simulink model "mrefrobotarm_modified_previous_y_previous_u_previous_ref_Thao"  (R2018b)
settings: Solver=FixedStepAuto  StartTime=0.0  StopTime=10  RelTol=1e-3  AbsTol=1e-6
undefined symbols (not defined in the file or in its folder): sfunxy2
libraries: neural x668, simulink x1
(part 11 of 21)

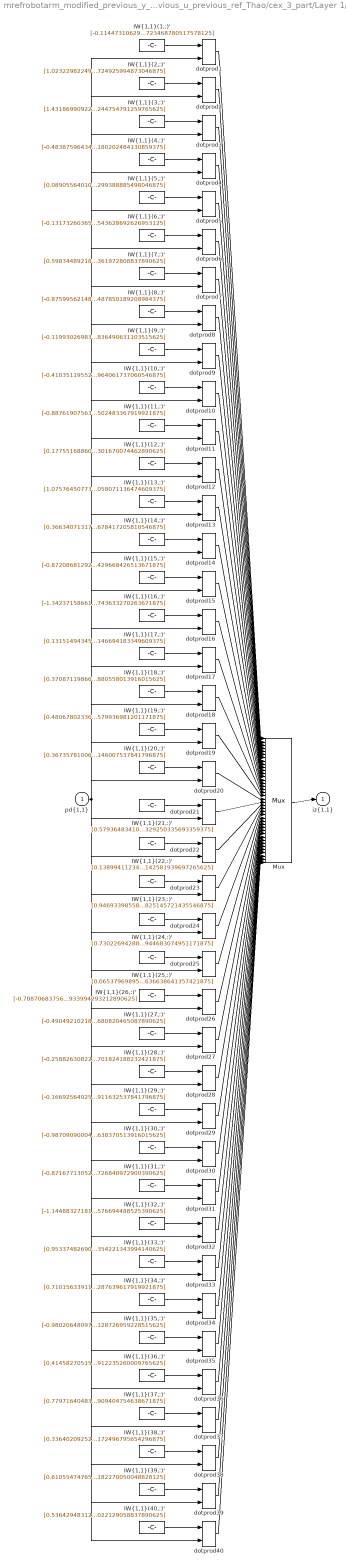
== system mrefrobotarm_modified_previous_y_previous_u_previous_ref_Thao/cex_3_part/Layer 1/IW{1,1} ==
  "pd{1,1}" : Inport  PortDimensions=10
      mask Display: e = 0.06;c1 = [120 230 180]/255;c2 = ([120 230 180]+0)/(256+128);c3 = ([120 230 180]+128)/(256+128);patch([0 1 1 0],[0 0 1 1],c1);patch([0 1 1 1-e 1-e 0+e],[0 0 1 1-e 0+e 0+e],c2);patch([0 0 1 1-e 0+e 0+e],[0 1 1 1-e 1-e 0+e],c3);plot([0 1 1 0 0],[0 0 1 1 0]);
  "IW{1,1}(1,:)'" : Constant  Value=[-0.11447310629155120487165930853734607808291912078857421875;1.4698726288777439474841912669944576919078826904296875;-0.1723351665624642536922550561939715407788753509521484375;0.06363633275744169648380221815386903472244739532470703125;-0.5064381225659226881674612741335295140743255615234375;-0.87026544298500951857278096213121898472309112548828125;-0.05463414776289564345201910100513487122952938079833984375;-1.13665173088892235142566278227604925632476806640625;0.268135298745105721263115583496983163058757781982421875;0.80221792322600216085248803210561163723468780517578125]
      mask Display: e = 0.06;c1 = [120 150 230]/255;c2 = ([120 150 230]+0)/383;c3 = ([120 150 230]+128)/383;patch([0 1 1 0],[0 0 1 1],c1);patch([0 1 1 1-e 1-e 0+e],[0 0 1 1-e 0+e 0+e],c2);patch([0 0 1 1-e 0+e 0+e],[0 1 1 1-e 1-e 0+e],c3);plot([0 1 1 0 0],[0 0 1 1 0]);disp('Weights');
  "IW{1,1}(10,:)'" : Constant  Value=[-0.41035119552119725394589977440773509442806243896484375;0.379787039117026992141035179884056560695171356201171875;-0.6683306949706373512043455775710754096508026123046875;-0.554820790867510016397545768995769321918487548828125;-0.71829482967000668480750391609035432338714599609375;0.447818372430159594710374904025229625403881072998046875;-0.55799752266937974187754889499046839773654937744140625;-0.379991668177938557438011457634274847805500030517578125;-0.340403705678418655455885755145573057234287261962890625;0.8973758576824291122164822809281758964061737060546875]
      mask Display: e = 0.06;c1 = [120 150 230]/255;c2 = ([120 150 230]+0)/383;c3 = ([120 150 230]+128)/383;patch([0 1 1 0],[0 0 1 1],c1);patch([0 1 1 1-e 1-e 0+e],[0 0 1 1-e 0+e 0+e],c2);patch([0 0 1 1-e 0+e 0+e],[0 1 1 1-e 1-e 0+e],c3);plot([0 1 1 0 0],[0 0 1 1 0]);disp('Weights');
  "IW{1,1}(11,:)'" : Constant  Value=[-0.8876190756363431244579942358541302382946014404296875;-1.025355338770573165874111509765498340129852294921875;0.1069134658050685526831102833966724574565887451171875;0.97378772065178031969168159776018001139163970947265625;-0.499558978367755146532402932280092500150203704833984375;-0.6707411879199665083461923131835646927356719970703125;-0.45046584360111163736206663088523782789707183837890625;0.415682749022733333266188537891139276325702667236328125;0.50981038413725221492001082879141904413700103759765625;-0.1924767238865232321654019642664934508502483367919921875]
      mask Display: e = 0.06;c1 = [120 150 230]/255;c2 = ([120 150 230]+0)/383;c3 = ([120 150 230]+128)/383;patch([0 1 1 0],[0 0 1 1],c1);patch([0 1 1 1-e 1-e 0+e],[0 0 1 1-e 0+e 0+e],c2);patch([0 0 1 1-e 0+e 0+e],[0 1 1 1-e 1-e 0+e],c3);plot([0 1 1 0 0],[0 0 1 1 0]);disp('Weights');
  "IW{1,1}(12,:)'" : Constant  Value=[0.177551688602920088033698675644700415432453155517578125;0.59145549863474300433807684385101310908794403076171875;-0.9027361748370814620301416653092019259929656982421875;0.70169416622816183082278485017013736069202423095703125;0.2632759672114854954116935914498753845691680908203125;0.392263699137575139186395745127811096608638763427734375;-0.444286429846018904310511743460665456950664520263671875;0.81245600109735327531979010018403641879558563232421875;-0.125222673969303255336882330084335990250110626220703125;0.0723812960570092978063172495239996351301670074462890625]
      mask Display: e = 0.06;c1 = [120 150 230]/255;c2 = ([120 150 230]+0)/383;c3 = ([120 150 230]+128)/383;patch([0 1 1 0],[0 0 1 1],c1);patch([0 1 1 1-e 1-e 0+e],[0 0 1 1-e 0+e 0+e],c2);patch([0 0 1 1-e 0+e 0+e],[0 1 1 1-e 1-e 0+e],c3);plot([0 1 1 0 0],[0 0 1 1 0]);disp('Weights');
  "IW{1,1}(13,:)'" : Constant  Value=[1.075764507733037333991887862794101238250732421875;-1.3033773750926440637698533464572392404079437255859375;0.06075593969214491962826940607556025497615337371826171875;0.077854453348255248101850156672298908233642578125;1.035365473561901783483563121990300714969635009765625;0.1045584350120265237915617717590066604316234588623046875;0.7663010865217769751467358219088055193424224853515625;0.5452525161551189381015092294546775519847869873046875;0.413026884388541237758118995770928449928760528564453125;0.23524197353400244647758654537028633058071136474609375]
      mask Display: e = 0.06;c1 = [120 150 230]/255;c2 = ([120 150 230]+0)/383;c3 = ([120 150 230]+128)/383;patch([0 1 1 0],[0 0 1 1],c1);patch([0 1 1 1-e 1-e 0+e],[0 0 1 1-e 0+e 0+e],c2);patch([0 0 1 1-e 0+e 0+e],[0 1 1 1-e 1-e 0+e],c3);plot([0 1 1 0 0],[0 0 1 1 0]);disp('Weights');
  "IW{1,1}(14,:)'" : Constant  Value=[0.366340713170913823137908593707834370434284210205078125;1.2545048824242097662562400728347711265087127685546875;-0.70126407125889678173535912719671614468097686767578125;-0.93088000136838722209375873717362992465496063232421875;-1.3149276252417114729809100026614032685756683349609375;1.01996655966251292824154006666503846645355224609375;0.27015749789315057771688088905648328363895416259765625;-0.5181576267080554298871675200643949210643768310546875;-0.09501464055484017123820450478888233192265033721923828125;1.0390900711406725331897860087337903678417205810546875]
      mask Display: e = 0.06;c1 = [120 150 230]/255;c2 = ([120 150 230]+0)/383;c3 = ([120 150 230]+128)/383;patch([0 1 1 0],[0 0 1 1],c1);patch([0 1 1 1-e 1-e 0+e],[0 0 1 1-e 0+e 0+e],c2);patch([0 0 1 1-e 0+e 0+e],[0 1 1 1-e 1-e 0+e],c3);plot([0 1 1 0 0],[0 0 1 1 0]);disp('Weights');
  "IW{1,1}(15,:)'" : Constant  Value=[-0.872086812929913524072844666079618036746978759765625;-0.303781258782407526108926276720012538135051727294921875;0.486042381521637256724943654262460768222808837890625;0.782441776717015979869529473944567143917083740234375;-0.1593782772753068732729531120639876462519168853759765625;0.1910372526839741735837918668039492331445217132568359375;0.354614546969915289675867597907199524343013763427734375;0.1656581200606266346397887900820933282375335693359375;-0.1446041112868961253656863163996604271233081817626953125;-0.92271215288813379640231460143695585429668426513671875]
      mask Display: e = 0.06;c1 = [120 150 230]/255;c2 = ([120 150 230]+0)/383;c3 = ([120 150 230]+128)/383;patch([0 1 1 0],[0 0 1 1],c1);patch([0 1 1 1-e 1-e 0+e],[0 0 1 1-e 0+e 0+e],c2);patch([0 0 1 1-e 0+e 0+e],[0 1 1 1-e 1-e 0+e],c3);plot([0 1 1 0 0],[0 0 1 1 0]);disp('Weights');
  "IW{1,1}(16,:)'" : Constant  Value=[-1.34237158661025457462301346822641789913177490234375;0.1745538377053377221415075837285257875919342041015625;0.08691722019173896141008839322239509783685207366943359375;0.14000144059391528283953221034607850015163421630859375;1.325323485870708584144495034706778824329376220703125;0.199762829956828202870866562079754658043384552001953125;0.53617616368730025566691210769931785762310028076171875;1.017650209419478368744194085593335330486297607421875;-0.4660995020663083465706222341395914554595947265625;0.73615171778669274971207414637319743633270263671875]
      mask Display: e = 0.06;c1 = [120 150 230]/255;c2 = ([120 150 230]+0)/383;c3 = ([120 150 230]+128)/383;patch([0 1 1 0],[0 0 1 1],c1);patch([0 1 1 1-e 1-e 0+e],[0 0 1 1-e 0+e 0+e],c2);patch([0 0 1 1-e 0+e 0+e],[0 1 1 1-e 1-e 0+e],c3);plot([0 1 1 0 0],[0 0 1 1 0]);disp('Weights');
  "IW{1,1}(17,:)'" : Constant  Value=[0.131514943452044674732093199054361321032047271728515625;0.86639289951866793604295935438130982220172882080078125;-0.72313729426715911419165649931528605520725250244140625;-1.1007955833634472941895410258439369499683380126953125;0.254690082949332374795403666212223470211029052734375;1.0086488328542049242031453104573301970958709716796875;0.0653956094404145316101306661948910914361476898193359375;-0.9184143325747744501796887561795301735401153564453125;0.2139545159164624454906089567884919233620166778564453125;-0.0497034786373153902871990794665180146694183349609375]
      mask Display: e = 0.06;c1 = [120 150 230]/255;c2 = ([120 150 230]+0)/383;c3 = ([120 150 230]+128)/383;patch([0 1 1 0],[0 0 1 1],c1);patch([0 1 1 1-e 1-e 0+e],[0 0 1 1-e 0+e 0+e],c2);patch([0 0 1 1-e 0+e 0+e],[0 1 1 1-e 1-e 0+e],c3);plot([0 1 1 0 0],[0 0 1 1 0]);disp('Weights');
  "IW{1,1}(18,:)'" : Constant  Value=[0.3708711986661497039818868870497681200504302978515625;0.7726639588684605097768098858068697154521942138671875;0.89188092512784322707375395111739635467529296875;-0.424566172674542385845342096217791549861431121826171875;-0.037912512550740677663707600686393561773002147674560546875;0.445005878596550441539392295453581027686595916748046875;-0.0086656709681872980122196992169847362674772739410400390625;0.450452395630884516730674249629373662173748016357421875;0.5326472508113422321684993221424520015716552734375;-0.69674411710658346041924460223526693880558013916015625]
      mask Display: e = 0.06;c1 = [120 150 230]/255;c2 = ([120 150 230]+0)/383;c3 = ([120 150 230]+128)/383;patch([0 1 1 0],[0 0 1 1],c1);patch([0 1 1 1-e 1-e 0+e],[0 0 1 1-e 0+e 0+e],c2);patch([0 0 1 1-e 0+e 0+e],[0 1 1 1-e 1-e 0+e],c3);plot([0 1 1 0 0],[0 0 1 1 0]);disp('Weights');
  "IW{1,1}(19,:)'" : Constant  Value=[0.480678023364515760729176463428302668035030364990234375;0.92052968620031638824485753502813167870044708251953125;-0.5639841933659950345969491536379791796207427978515625;0.80826204135619705848370131207047961652278900146484375;0.87363147720026945730609213569550774991512298583984375;0.348510708652358947023941482257214374840259552001953125;0.28549287950379664824396286348928697407245635986328125;-0.313463044792744505162573886991594918072223663330078125;1.07366761594383586242429373669438064098358154296875;-0.1598076346574494877028627115578274242579936981201171875]
      mask Display: e = 0.06;c1 = [120 150 230]/255;c2 = ([120 150 230]+0)/383;c3 = ([120 150 230]+128)/383;patch([0 1 1 0],[0 0 1 1],c1);patch([0 1 1 1-e 1-e 0+e],[0 0 1 1-e 0+e 0+e],c2);patch([0 0 1 1-e 0+e 0+e],[0 1 1 1-e 1-e 0+e],c3);plot([0 1 1 0 0],[0 0 1 1 0]);disp('Weights');
  "IW{1,1}(2,:)'" : Constant  Value=[1.023229822492787821630599864874966442584991455078125;0.360014655376229952832289882280747406184673309326171875;0.50752088515731375029105265639373101294040679931640625;0.200233829267601304291446240313234739005565643310546875;1.136229259214101450226053202641196548938751220703125;-0.75286639627510421046707733694347552955150604248046875;0.78621498258449429297201049848808906972408294677734375;0.63666905569844434165105440115439705550670623779296875;-0.0718307003896297702194573275846778415143489837646484375;0.47372532853303706001923956137034110724925994873046875]
      mask Display: e = 0.06;c1 = [120 150 230]/255;c2 = ([120 150 230]+0)/383;c3 = ([120 150 230]+128)/383;patch([0 1 1 0],[0 0 1 1],c1);patch([0 1 1 1-e 1-e 0+e],[0 0 1 1-e 0+e 0+e],c2);patch([0 0 1 1-e 0+e 0+e],[0 1 1 1-e 1-e 0+e],c3);plot([0 1 1 0 0],[0 0 1 1 0]);disp('Weights');
  "IW{1,1}(20,:)'" : Constant  Value=[0.36735781006335066489754126450861804187297821044921875;0.6846723849940870021413275026134215295314788818359375;-0.898232615997065497737139594391919672489166259765625;-1.005037189194012636761499379645101726055145263671875;-0.033184850310548401342014557258153217844665050506591796875;0.61255686246330098843060341096133925020694732666015625;1.1804909974660677818292242591269314289093017578125;-0.42085789393468842067846935606212355196475982666015625;0.52684594563863085259214358302415348589420318603515625;-0.300991274102481998209412950018304400146007537841796875]
      mask Display: e = 0.06;c1 = [120 150 230]/255;c2 = ([120 150 230]+0)/383;c3 = ([120 150 230]+128)/383;patch([0 1 1 0],[0 0 1 1],c1);patch([0 1 1 1-e 1-e 0+e],[0 0 1 1-e 0+e 0+e],c2);patch([0 0 1 1-e 0+e 0+e],[0 1 1 1-e 1-e 0+e],c3);plot([0 1 1 0 0],[0 0 1 1 0]);disp('Weights');
  "IW{1,1}(21,:)'" : Constant  Value=[0.579364834101031789259650395251810550689697265625;0.68869445913839200112960270416806451976299285888671875;0.40311996786962278616073263037833385169506072998046875;0.58457664968583300524329615655005909502506256103515625;0.81869531744760737357324842378147877752780914306640625;-1.035458973817988681531687689130194485187530517578125;-0.63548022585192642797125017750659026205539703369140625;0.458258309449441070260178321404964663088321685791015625;-0.20436707588377645006261218441068194806575775146484375;0.52439609974291412353153418735018931329250335693359375]
      mask Display: e = 0.06;c1 = [120 150 230]/255;c2 = ([120 150 230]+0)/383;c3 = ([120 150 230]+128)/383;patch([0 1 1 0],[0 0 1 1],c1);patch([0 1 1 1-e 1-e 0+e],[0 0 1 1-e 0+e 0+e],c2);patch([0 0 1 1-e 0+e 0+e],[0 1 1 1-e 1-e 0+e],c3);plot([0 1 1 0 0],[0 0 1 1 0]);disp('Weights');
  "IW{1,1}(22,:)'" : Constant  Value=[0.1389941123461821692597339961139368824660778045654296875;0.7697497284234093850585622931248508393764495849609375;-0.69868899535862938332542171337991021573543548583984375;-0.1464612409619554800332963395703700371086597442626953125;-0.9217585889346635585894773612380959093570709228515625;-0.81337527403198872644196626424673013389110565185546875;0.334544050732859699071042314244550652801990509033203125;-1.226150884523554029925662689493037760257720947265625;-0.08119914826178963040970160136566846631467342376708984375;0.2650476076761754118393810131237842142581939697265625]
      mask Display: e = 0.06;c1 = [120 150 230]/255;c2 = ([120 150 230]+0)/383;c3 = ([120 150 230]+128)/383;patch([0 1 1 0],[0 0 1 1],c1);patch([0 1 1 1-e 1-e 0+e],[0 0 1 1-e 0+e 0+e],c2);patch([0 0 1 1-e 0+e 0+e],[0 1 1 1-e 1-e 0+e],c3);plot([0 1 1 0 0],[0 0 1 1 0]);disp('Weights');
  "IW{1,1}(23,:)'" : Constant  Value=[0.94693398558723684832472144989878870546817779541015625;0.93810260377214926830191643603029660880565643310546875;-0.416295931351030545908287194833974353969097137451171875;0.71022710849672476829397282926947809755802154541015625;-0.07271652756315809262854799044362152926623821258544921875;0.85947723902092276748732047053636051714420318603515625;-0.5342648617709799818698002127348445355892181396484375;0.295986597537863327378460098771029151976108551025390625;-0.107446552770858405612131036832579411566257476806640625;1.064860279315108737563377871992997825145721435546875]
      mask Display: e = 0.06;c1 = [120 150 230]/255;c2 = ([120 150 230]+0)/383;c3 = ([120 150 230]+128)/383;patch([0 1 1 0],[0 0 1 1],c1);patch([0 1 1 1-e 1-e 0+e],[0 0 1 1-e 0+e 0+e],c2);patch([0 0 1 1-e 0+e 0+e],[0 1 1 1-e 1-e 0+e],c3);plot([0 1 1 0 0],[0 0 1 1 0]);disp('Weights');
  "IW{1,1}(24,:)'" : Constant  Value=[0.73022694288870315659778498229570686817169189453125;0.048085778005342916241460216042469255626201629638671875;0.361376798420908362796666324356920085847377777099609375;1.0616565820681496123967235689633525907993316650390625;-0.11901986901194673562631720642457366921007633209228515625;-0.91563209752461494073116909930831752717494964599609375;-0.69473400065113699586305529010132886469364166259765625;0.363295935990913754221054432491655461490154266357421875;0.360477705297992667698991908764583058655261993408203125;-0.9688106558803084578102016166667453944683074951171875]
      mask Display: e = 0.06;c1 = [120 150 230]/255;c2 = ([120 150 230]+0)/383;c3 = ([120 150 230]+128)/383;patch([0 1 1 0],[0 0 1 1],c1);patch([0 1 1 1-e 1-e 0+e],[0 0 1 1-e 0+e 0+e],c2);patch([0 0 1 1-e 0+e 0+e],[0 1 1 1-e 1-e 0+e],c3);plot([0 1 1 0 0],[0 0 1 1 0]);disp('Weights');
  "IW{1,1}(25,:)'" : Constant  Value=[0.06537969895563856825848603193662711419165134429931640625;-0.74425177721775892525357676277053542435169219970703125;0.96676618935224312156861969924648292362689971923828125;-1.1788259854350446875770330734667368233203887939453125;0.166660640443120178222358163111493922770023345947265625;0.7552338671992175900271604405133984982967376708984375;-0.23659770418445569273302453439100645482540130615234375;-0.84178927100927525284390640081255696713924407958984375;-0.2197799957382577940023793416912667453289031982421875;-0.09291332901493314089247377296487684361636638641357421875]
      mask Display: e = 0.06;c1 = [120 150 230]/255;c2 = ([120 150 230]+0)/383;c3 = ([120 150 230]+128)/383;patch([0 1 1 0],[0 0 1 1],c1);patch([0 1 1 1-e 1-e 0+e],[0 0 1 1-e 0+e 0+e],c2);patch([0 0 1 1-e 0+e 0+e],[0 1 1 1-e 1-e 0+e],c3);plot([0 1 1 0 0],[0 0 1 1 0]);disp('Weights');
  "IW{1,1}(26,:)'" : Constant  Value=[-0.78870683756448567436336816172115504741668701171875;0.59214368731254463096291829060646705329418182373046875;0.68284740354832218489633532954030670225620269775390625;-0.9010509244307172149746065770159475505352020263671875;0.748179715690247437720472589717246592044830322265625;0.3793116045733027075215204604319296777248382568359375;0.211379014616436933238219353370368480682373046875;0.68539438327457535837794466715422458946704864501953125;0.0168086311280647403287868968391194357536733150482177734375;0.9444837524589113630923975506448186933994293212890625]
      mask Display: e = 0.06;c1 = [120 150 230]/255;c2 = ([120 150 230]+0)/383;c3 = ([120 150 230]+128)/383;patch([0 1 1 0],[0 0 1 1],c1);patch([0 1 1 1-e 1-e 0+e],[0 0 1 1-e 0+e 0+e],c2);patch([0 0 1 1-e 0+e 0+e],[0 1 1 1-e 1-e 0+e],c3);plot([0 1 1 0 0],[0 0 1 1 0]);disp('Weights');
  "IW{1,1}(27,:)'" : Constant  Value=[-0.490492102187102874122359708053409121930599212646484375;-0.28299615554411428064440769958309829235076904296875;0.84104621798512180230744661457720212638378143310546875;-0.54478269880424290416698340777656994760036468505859375;0.49715034809935121362656218479969538748264312744140625;-0.671561590720024081946348815108649432659149169921875;0.1776535023858118178541332099484861828386783599853515625;0.1223916850472323292198240096695371903479099273681640625;1.005040312956411607814288800000213086605072021484375;-0.527848866809601080518632443272508680820465087890625]
      mask Display: e = 0.06;c1 = [120 150 230]/255;c2 = ([120 150 230]+0)/383;c3 = ([120 150 230]+128)/383;patch([0 1 1 0],[0 0 1 1],c1);patch([0 1 1 1-e 1-e 0+e],[0 0 1 1-e 0+e 0+e],c2);patch([0 0 1 1-e 0+e 0+e],[0 1 1 1-e 1-e 0+e],c3);plot([0 1 1 0 0],[0 0 1 1 0]);disp('Weights');
  "IW{1,1}(28,:)'" : Constant  Value=[-0.258826308223806478281403542496263980865478515625;-1.0210882986596903077014530936139635741710662841796875;0.46664800819570484424758660679799504578113555908203125;-0.88163202623709946426089345550280995666980743408203125;-0.617805738329396003649662816314958035945892333984375;-0.24228190721330944423783648744574747979640960693359375;-0.8551741086002586644809753124718554317951202392578125;-0.38921322699798455158060050962376408278942108154296875;-0.432604691806382835039812562172301113605499267578125;-0.252551012942012043094308637591893784701824188232421875]
      mask Display: e = 0.06;c1 = [120 150 230]/255;c2 = ([120 150 230]+0)/383;c3 = ([120 150 230]+128)/383;patch([0 1 1 0],[0 0 1 1],c1);patch([0 1 1 1-e 1-e 0+e],[0 0 1 1-e 0+e 0+e],c2);patch([0 0 1 1-e 0+e 0+e],[0 1 1 1-e 1-e 0+e],c3);plot([0 1 1 0 0],[0 0 1 1 0]);disp('Weights');
  "IW{1,1}(29,:)'" : Constant  Value=[-0.1669256402556720531027423248815466649830341339111328125;0.443796693399950037406398450912092812359333038330078125;0.5283293737470582396298368621501140296459197998046875;-0.279978607770516918495928848642506636679172515869140625;0.6096342129880618632142841306631453335285186767578125;0.76092861455241489476719607409904710948467254638671875;-1.24926264460642943987522812676616013050079345703125;0.435208015196196174034781734007992781698703765869140625;-0.57445794996099153184587748910416848957538604736328125;0.86080824776438180645499187448876909911632537841796875]
      mask Display: e = 0.06;c1 = [120 150 230]/255;c2 = ([120 150 230]+0)/383;c3 = ([120 150 230]+128)/383;patch([0 1 1 0],[0 0 1 1],c1);patch([0 1 1 1-e 1-e 0+e],[0 0 1 1-e 0+e 0+e],c2);patch([0 0 1 1-e 0+e 0+e],[0 1 1 1-e 1-e 0+e],c3);plot([0 1 1 0 0],[0 0 1 1 0]);disp('Weights');
  "IW{1,1}(3,:)'" : Constant  Value=[1.431869909221603620608220808207988739013671875;-1.0829285977574183430505172509583644568920135498046875;0.284110948167406174302840327072772197425365447998046875;-0.0908891676367490630727985490011633373796939849853515625;-0.71644139254706384889459513942711055278778076171875;0.9394257302715602886422630035667680203914642333984375;-0.006340994204176671200645643011739593930542469024658203125;0.96520723140826414354620510493987239897251129150390625;-0.80121031571460343823076755143119953572750091552734375;0.125751024592712090655055590104893781244754791259765625]
      mask Display: e = 0.06;c1 = [120 150 230]/255;c2 = ([120 150 230]+0)/383;c3 = ([120 150 230]+128)/383;patch([0 1 1 0],[0 0 1 1],c1);patch([0 1 1 1-e 1-e 0+e],[0 0 1 1-e 0+e 0+e],c2);patch([0 0 1 1-e 0+e 0+e],[0 1 1 1-e 1-e 0+e],c3);plot([0 1 1 0 0],[0 0 1 1 0]);disp('Weights');
  "IW{1,1}(30,:)'" : Constant  Value=[-0.98709090004929589401427847406012006103992462158203125;-0.574921453538869808852496134932152926921844482421875;0.98761523674588180821132255005068145692348480224609375;0.788637145693480423602750306599773466587066650390625;-0.740764059382627237937413156032562255859375;0.80848404746890489835919879624270834028720855712890625;-1.234937646145773282313484742189757525920867919921875;-0.132070256945421959926534327678382396697998046875;0.93884515207616081600150437225238420069217681884765625;0.6474367534507250443454040578217245638370513916015625]
      mask Display: e = 0.06;c1 = [120 150 230]/255;c2 = ([120 150 230]+0)/383;c3 = ([120 150 230]+128)/383;patch([0 1 1 0],[0 0 1 1],c1);patch([0 1 1 1-e 1-e 0+e],[0 0 1 1-e 0+e 0+e],c2);patch([0 0 1 1-e 0+e 0+e],[0 1 1 1-e 1-e 0+e],c3);plot([0 1 1 0 0],[0 0 1 1 0]);disp('Weights');
  "IW{1,1}(31,:)'" : Constant  Value=[-0.8716771305245620826696040239767171442508697509765625;-0.45752045805780727771860938446479849517345428466796875;-0.59421933988957131855812576759490184485912322998046875;0.30020948661724522477101118056452833116054534912109375;0.63894685369801129670719319619820453226566314697265625;0.313065408721107940603900487985811196267604827880859375;-0.51252670466233796187083271433948539197444915771484375;-0.5004001117209979643263295656652189791202545166015625;1.0772116853349036347253786516375839710235595703125;-0.172318440890303126167282243841327726840972900390625]
      mask Display: e = 0.06;c1 = [120 150 230]/255;c2 = ([120 150 230]+0)/383;c3 = ([120 150 230]+128)/383;patch([0 1 1 0],[0 0 1 1],c1);patch([0 1 1 1-e 1-e 0+e],[0 0 1 1-e 0+e 0+e],c2);patch([0 0 1 1-e 0+e 0+e],[0 1 1 1-e 1-e 0+e],c3);plot([0 1 1 0 0],[0 0 1 1 0]);disp('Weights');
  "IW{1,1}(32,:)'" : Constant  Value=[-1.1448832718126451535312071428052149713039398193359375;0.6633963684966663887365712071186862885951995849609375;0.609383247785491022341375355608761310577392578125;-0.715808214472330117672527194372378289699554443359375;-1.350495171029303609344651704304851591587066650390625;-0.350264501467584865590509934918372891843318939208984375;-0.185317616157214093419725031708367168903350830078125;-0.88932181315658243025978890727856196463108062744140625;-0.67848419917436986192882386603741906583309173583984375;0.66262782521406649038908653892576694488525390625]
      mask Display: e = 0.06;c1 = [120 150 230]/255;c2 = ([120 150 230]+0)/383;c3 = ([120 150 230]+128)/383;patch([0 1 1 0],[0 0 1 1],c1);patch([0 1 1 1-e 1-e 0+e],[0 0 1 1-e 0+e 0+e],c2);patch([0 0 1 1-e 0+e 0+e],[0 1 1 1-e 1-e 0+e],c3);plot([0 1 1 0 0],[0 0 1 1 0]);disp('Weights');
  "IW{1,1}(33,:)'" : Constant  Value=[0.95337482690746966351724722699145786464214324951171875;-0.9996434333293786611562836696975864470005035400390625;-0.58116139181709847161272364246542565524578094482421875;-0.3238044768967520692370953838690184056758880615234375;0.7482564483354341433596346178092062473297119140625;-0.063883302415352838377060606944723986089229583740234375;-0.89121478895607186831995250031468458473682403564453125;-0.5689491350695068394571762837585993111133575439453125;-0.489426654220092516300866236633737571537494659423828125;0.76200280191338976010229089297354221343994140625]
      mask Display: e = 0.06;c1 = [120 150 230]/255;c2 = ([120 150 230]+0)/383;c3 = ([120 150 230]+128)/383;patch([0 1 1 0],[0 0 1 1],c1);patch([0 1 1 1-e 1-e 0+e],[0 0 1 1-e 0+e 0+e],c2);patch([0 0 1 1-e 0+e 0+e],[0 1 1 1-e 1-e 0+e],c3);plot([0 1 1 0 0],[0 0 1 1 0]);disp('Weights');
  "IW{1,1}(34,:)'" : Constant  Value=[0.710156339117125501303462442592717707157135009765625;-0.2706694720472118120824234210886061191558837890625;-1.0981648407871753558850969056948088109493255615234375;-0.93349618659047595148336995407589711248874664306640625;-0.32271336598055755384706344557343982160091400146484375;-0.67481838191983778418858719305717386305332183837890625;-0.514094431635296000848711628350429236888885498046875;-0.35718986061501756257285933315870352089405059814453125;0.8114450781619007013745203948928974568843841552734375;0.5165824011811401827998224689508788287639617919921875]
      mask Display: e = 0.06;c1 = [120 150 230]/255;c2 = ([120 150 230]+0)/383;c3 = ([120 150 230]+128)/383;patch([0 1 1 0],[0 0 1 1],c1);patch([0 1 1 1-e 1-e 0+e],[0 0 1 1-e 0+e 0+e],c2);patch([0 0 1 1-e 0+e 0+e],[0 1 1 1-e 1-e 0+e],c3);plot([0 1 1 0 0],[0 0 1 1 0]);disp('Weights');
  "IW{1,1}(35,:)'" : Constant  Value=[-0.9802064809722705884809101917198859155178070068359375;-0.75883472139506469300584967641043476760387420654296875;0.256199983711767054206376315050874836742877960205078125;0.70933174537725440789159847554401494562625885009765625;1.286194324249188891684525515302084386348724365234375;-1.249366492046050769459952789475210011005401611328125;-0.417243569265245695110166934682638384401798248291015625;-0.614031022376110069416199621628038585186004638671875;0.1954842559935171253382435452294885180890560150146484375;0.14922243704243653983354533920646645128726959228515625]
      mask Display: e = 0.06;c1 = [120 150 230]/255;c2 = ([120 150 230]+0)/383;c3 = ([120 150 230]+128)/383;patch([0 1 1 0],[0 0 1 1],c1);patch([0 1 1 1-e 1-e 0+e],[0 0 1 1-e 0+e 0+e],c2);patch([0 0 1 1-e 0+e 0+e],[0 1 1 1-e 1-e 0+e],c3);plot([0 1 1 0 0],[0 0 1 1 0]);disp('Weights');
  "IW{1,1}(36,:)'" : Constant  Value=[0.414582705158955178159629895162652246654033660888671875;0.50023649309523821049339176170178689062595367431640625;0.35735462983669441516809683889732696115970611572265625;0.84040612720998819629159015676123090088367462158203125;0.426695431620777110293118994377437047660350799560546875;0.1238275402082783804846854991410509683191776275634765625;0.81971070288723002494890579328057356178760528564453125;-0.2377061934897990724824268227166612632572650909423828125;0.983973589538960080602691959938965737819671630859375;-1.157225452410207910958206412033177912235260009765625]
      mask Display: e = 0.06;c1 = [120 150 230]/255;c2 = ([120 150 230]+0)/383;c3 = ([120 150 230]+128)/383;patch([0 1 1 0],[0 0 1 1],c1);patch([0 1 1 1-e 1-e 0+e],[0 0 1 1-e 0+e 0+e],c2);patch([0 0 1 1-e 0+e 0+e],[0 1 1 1-e 1-e 0+e],c3);plot([0 1 1 0 0],[0 0 1 1 0]);disp('Weights');
  "IW{1,1}(37,:)'" : Constant  Value=[0.7797164048356195475975027875392697751522064208984375;0.32596768621032079504828971039387397468090057373046875;0.096769847541164299986604646619525738060474395751953125;0.923797525894631821330449383822269737720489501953125;-0.26619991333689940748996605179854668676853179931640625;1.0828906280626664493382804721477441489696502685546875;-0.353496680686303410556803328290698118507862091064453125;0.81390378005917696224713608899037353694438934326171875;0.34502388372655190540427838641335256397724151611328125;0.756185963111658310253915260545909404754638671875]
      mask Display: e = 0.06;c1 = [120 150 230]/255;c2 = ([120 150 230]+0)/383;c3 = ([120 150 230]+128)/383;patch([0 1 1 0],[0 0 1 1],c1);patch([0 1 1 1-e 1-e 0+e],[0 0 1 1-e 0+e 0+e],c2);patch([0 0 1 1-e 0+e 0+e],[0 1 1 1-e 1-e 0+e],c3);plot([0 1 1 0 0],[0 0 1 1 0]);disp('Weights');
  "IW{1,1}(38,:)'" : Constant  Value=[0.336402092525067641926028727539232932031154632568359375;0.32445693985996337804778022473328746855258941650390625;-0.27547690707819494360109047192963771522045135498046875;-0.035685155755691540246932191848827642388641834259033203125;-0.1924028740524797165267756327011738903820514678955078125;1.40500614577392202164674017694778740406036376953125;0.232225589660242537348722180468030273914337158203125;1.1698446174636993877271606834256090223789215087890625;-0.3305143996269723771774806664325296878814697265625;-0.0307955824755770206369032138127295183949172496795654296875]
      mask Display: e = 0.06;c1 = [120 150 230]/255;c2 = ([120 150 230]+0)/383;c3 = ([120 150 230]+128)/383;patch([0 1 1 0],[0 0 1 1],c1);patch([0 1 1 1-e 1-e 0+e],[0 0 1 1-e 0+e 0+e],c2);patch([0 0 1 1-e 0+e 0+e],[0 1 1 1-e 1-e 0+e],c3);plot([0 1 1 0 0],[0 0 1 1 0]);disp('Weights');
  "IW{1,1}(39,:)'" : Constant  Value=[0.61055474765612094412148280753172002732753753662109375;-0.1905274841282655617913377454897272400557994842529296875;-0.050964228009610083869329599792763474397361278533935546875;-0.6172492952399057930534809202072210609912872314453125;-0.541132777055141733768550693639554083347320556640625;0.69377595265419189640709873856394551694393157958984375;-0.58344798589655777476536968606524169445037841796875;0.2363636904125665794129673713541706092655658721923828125;0.1995627084764219072443580671460949815809726715087890625;-0.03323088703474126603953919811829109676182270050048828125]
      mask Display: e = 0.06;c1 = [120 150 230]/255;c2 = ([120 150 230]+0)/383;c3 = ([120 150 230]+128)/383;patch([0 1 1 0],[0 0 1 1],c1);patch([0 1 1 1-e 1-e 0+e],[0 0 1 1-e 0+e 0+e],c2);patch([0 0 1 1-e 0+e 0+e],[0 1 1 1-e 1-e 0+e],c3);plot([0 1 1 0 0],[0 0 1 1 0]);disp('Weights');
  "IW{1,1}(4,:)'" : Constant  Value=[-0.483875964345077125283722807580488733947277069091796875;1.4294021819731714817436341036227531731128692626953125;-0.303153199789456817558885859398287720978260040283203125;0.6419145304898652426572880358435213565826416015625;-1.9610237994277894824080021862755529582500457763671875;0.5238633373172987273136413932661525905132293701171875;-0.5113929129788135075074251290061511099338531494140625;-0.54187244687960200995036075255484320223331451416015625;0.2125665724778078302659167775345849804580211639404296875;0.310104598980188439494298791032633744180202484130859375]
      mask Display: e = 0.06;c1 = [120 150 230]/255;c2 = ([120 150 230]+0)/383;c3 = ([120 150 230]+128)/383;patch([0 1 1 0],[0 0 1 1],c1);patch([0 1 1 1-e 1-e 0+e],[0 0 1 1-e 0+e 0+e],c2);patch([0 0 1 1-e 0+e 0+e],[0 1 1 1-e 1-e 0+e],c3);plot([0 1 1 0 0],[0 0 1 1 0]);disp('Weights');
  "IW{1,1}(40,:)'" : Constant  Value=[0.53642948312383875730802174075506627559661865234375;-0.918510324537320510529525563470087945461273193359375;0.4951566506339604156750056063174270093441009521484375;-1.1186177745236929315097995640826411545276641845703125;0.05973584011020897921451222600808250717818737030029296875;-0.0653382230579835077133310505814733915030956268310546875;-0.1443357408137461994623862437947536818683147430419921875;-0.34541986358497644982179508588160388171672821044921875;1.148399778239722390793531303643248975276947021484375;-0.52504595413077803645052199499332346022129058837890625]
      mask Display: e = 0.06;c1 = [120 150 230]/255;c2 = ([120 150 230]+0)/383;c3 = ([120 150 230]+128)/383;patch([0 1 1 0],[0 0 1 1],c1);patch([0 1 1 1-e 1-e 0+e],[0 0 1 1-e 0+e 0+e],c2);patch([0 0 1 1-e 0+e 0+e],[0 1 1 1-e 1-e 0+e],c3);plot([0 1 1 0 0],[0 0 1 1 0]);disp('Weights');
  "IW{1,1}(5,:)'" : Constant  Value=[0.08905564010308440747731850706259137950837612152099609375;0.6750657336578853584541093368898145854473114013671875;0.76444002446765157987584871079889126121997833251953125;-0.76818370001505364985661117316340096294879913330078125;1.3528895341285871456449285687995143234729766845703125;-0.41807614315741525867764494250877760350704193115234375;-0.026367899404192651768852329041692428290843963623046875;0.017467804530305781895993533225919236429035663604736328125;-1.0102682741945383515513867678237147629261016845703125;0.33322752068363026278774441379937343299388885498046875]
      mask Display: e = 0.06;c1 = [120 150 230]/255;c2 = ([120 150 230]+0)/383;c3 = ([120 150 230]+128)/383;patch([0 1 1 0],[0 0 1 1],c1);patch([0 1 1 1-e 1-e 0+e],[0 0 1 1-e 0+e 0+e],c2);patch([0 0 1 1-e 0+e 0+e],[0 1 1 1-e 1-e 0+e],c3);plot([0 1 1 0 0],[0 0 1 1 0]);disp('Weights');
  "IW{1,1}(6,:)'" : Constant  Value=[-0.131732603650755619728585088523686863481998443603515625;0.018958868949519480651133562787435948848724365234375;0.93627818985862110157114557296154089272022247314453125;0.6197363090051635214905445536714978516101837158203125;0.66650024883545622156333365637692622840404510498046875;-0.118624990938835661591355119526269845664501190185546875;0.65136412215784911250437971830251626670360565185546875;-0.1787922059470858637819645764466258697211742401123046875;0.94205117033140339799501816742122173309326171875;-0.9434419869175034722985628832248039543628692626953125]
      mask Display: e = 0.06;c1 = [120 150 230]/255;c2 = ([120 150 230]+0)/383;c3 = ([120 150 230]+128)/383;patch([0 1 1 0],[0 0 1 1],c1);patch([0 1 1 1-e 1-e 0+e],[0 0 1 1-e 0+e 0+e],c2);patch([0 0 1 1-e 0+e 0+e],[0 1 1 1-e 1-e 0+e],c3);plot([0 1 1 0 0],[0 0 1 1 0]);disp('Weights');
  "IW{1,1}(7,:)'" : Constant  Value=[0.59834489218407493904550165098044089972972869873046875;-1.0722763448806349462216758183785714209079742431640625;-0.404456556970482328239313574158586561679840087890625;-0.48621331328340022803757847214001230895519256591796875;1.8919637028463480721285350227844901382923126220703125;-0.23618954779038070501684387636487372219562530517578125;0.027539004053715961106707510452906717546284198760986328125;-0.443386634518811717509123582203756086528301239013671875;0.044284048581706626779297408802449353970587253570556640625;-0.65838396534664733739106168286525644361972808837890625]
      mask Display: e = 0.06;c1 = [120 150 230]/255;c2 = ([120 150 230]+0)/383;c3 = ([120 150 230]+128)/383;patch([0 1 1 0],[0 0 1 1],c1);patch([0 1 1 1-e 1-e 0+e],[0 0 1 1-e 0+e 0+e],c2);patch([0 0 1 1-e 0+e 0+e],[0 1 1 1-e 1-e 0+e],c3);plot([0 1 1 0 0],[0 0 1 1 0]);disp('Weights');
  "IW{1,1}(8,:)'" : Constant  Value=[-0.8759956214844899502480757291777990758419036865234375;-0.68957728559488007391564678982831537723541259765625;-0.56571937693497442722900814260356128215789794921875;0.5365302359733259418561601705732755362987518310546875;-0.6096060411952597402063247500336728990077972412109375;-0.54503427877826216008116944067296572029590606689453125;0.491948017634882550641606258068350143730640411376953125;-0.879355439450711262594495565281249582767486572265625;-0.824521539487706345283868358819745481014251708984375;-1.1714334453650623313336609498946927487850189208984375]
      mask Display: e = 0.06;c1 = [120 150 230]/255;c2 = ([120 150 230]+0)/383;c3 = ([120 150 230]+128)/383;patch([0 1 1 0],[0 0 1 1],c1);patch([0 1 1 1-e 1-e 0+e],[0 0 1 1-e 0+e 0+e],c2);patch([0 0 1 1-e 0+e 0+e],[0 1 1 1-e 1-e 0+e],c3);plot([0 1 1 0 0],[0 0 1 1 0]);disp('Weights');
  "IW{1,1}(9,:)'" : Constant  Value=[-0.1199302698325285521097072205520817078649997711181640625;1.429733850212643542221258030622266232967376708984375;-0.296792982577691211165671347771422006189823150634765625;0.149719958454178903028974900735192932188510894775390625;-0.8840337365195962693320552716613747179508209228515625;0.90778542967060837920456606298102997243404388427734375;-0.07005205050979201875094304341473616659641265869140625;0.2597200075356493886857833786052651703357696533203125;0.9791926266214112661856461272691376507282257080078125;0.183746314348932016091708874228061176836490631103515625]
      mask Display: e = 0.06;c1 = [120 150 230]/255;c2 = ([120 150 230]+0)/383;c3 = ([120 150 230]+128)/383;patch([0 1 1 0],[0 0 1 1],c1);patch([0 1 1 1-e 1-e 0+e],[0 0 1 1-e 0+e 0+e],c2);patch([0 0 1 1-e 0+e 0+e],[0 1 1 1-e 1-e 0+e],c3);plot([0 1 1 0 0],[0 0 1 1 0]);disp('Weights');
  Mux : Mux  Inputs=40
      mask Display: e = 0.06;c1 = [120 150 230]/255;c2 = ([120 150 230]+0)/383;c3 = ([120 150 230]+128)/383;patch([0 1 1 0],[0 0 1 1],c1);patch([0 1 1 1-e 1-e 0+e],[0 0 1 1-e 0+e 0+e],c2);patch([0 0 1 1-e 0+e 0+e],[0 1 1 1-e 1-e 0+e],c3);plot([0 1 1 0 0],[0 0 1 1 0]);disp('Mux');
  dotprod{1..40} (40 alike) : neural/Weight Functions/dotprod
  "iz{1,1}" : Outport
      mask Display: e = 0.06;c1 = [120 230 180]/255;c2 = ([120 230 180]+0)/(256+128);c3 = ([120 230 180]+128)/(256+128);patch([0 1 1 0],[0 0 1 1],c1);patch([0 1 1 1-e 1-e 0+e],[0 0 1 1-e 0+e 0+e],c2);patch([0 0 1 1-e 0+e 0+e],[0 1 1 1-e 1-e 0+e],c3);plot([0 1 1 0 0],[0 0 1 1 0]);
  wires:
  "IW{1,1}(1,:)'"/1 -> dotprod1/1
  "pd{1,1}"/1 -> dotprod1/2, dotprod2/2, dotprod3/2, dotprod4/2, dotprod5/2, dotprod6/2, dotprod7/2, dotprod8/2, dotprod9/2, dotprod10/2, dotprod11/2, dotprod12/2, dotprod13/2, dotprod14/2, dotprod15/2, dotprod16/2, dotprod17/2, dotprod18/2, dotprod19/2, dotprod20/2, dotprod21/2, dotprod22/2, dotprod23/2, dotprod24/2, dotprod25/2, dotprod26/2, dotprod27/2, dotprod28/2, dotprod29/2, dotprod30/2, dotprod31/2, dotprod32/2, dotprod33/2, dotprod34/2, dotprod35/2, dotprod36/2, dotprod37/2, dotprod38/2, dotprod39/2, dotprod40/2
  dotprod1/1 -> Mux/1
  "IW{1,1}(2,:)'"/1 -> dotprod2/1
  dotprod2/1 -> Mux/2
  "IW{1,1}(3,:)'"/1 -> dotprod3/1
  dotprod3/1 -> Mux/3
  "IW{1,1}(4,:)'"/1 -> dotprod4/1
  dotprod4/1 -> Mux/4
  "IW{1,1}(5,:)'"/1 -> dotprod5/1
  dotprod5/1 -> Mux/5
  "IW{1,1}(6,:)'"/1 -> dotprod6/1
  dotprod6/1 -> Mux/6
  "IW{1,1}(7,:)'"/1 -> dotprod7/1
  dotprod7/1 -> Mux/7
  "IW{1,1}(8,:)'"/1 -> dotprod8/1
  dotprod8/1 -> Mux/8
  "IW{1,1}(9,:)'"/1 -> dotprod9/1
  dotprod9/1 -> Mux/9
  "IW{1,1}(10,:)'"/1 -> dotprod10/1
  dotprod10/1 -> Mux/10
  "IW{1,1}(11,:)'"/1 -> dotprod11/1
  dotprod11/1 -> Mux/11
  "IW{1,1}(12,:)'"/1 -> dotprod12/1
  dotprod12/1 -> Mux/12
  "IW{1,1}(13,:)'"/1 -> dotprod13/1
  dotprod13/1 -> Mux/13
  "IW{1,1}(14,:)'"/1 -> dotprod14/1
  dotprod14/1 -> Mux/14
  "IW{1,1}(15,:)'"/1 -> dotprod15/1
  dotprod15/1 -> Mux/15
  "IW{1,1}(16,:)'"/1 -> dotprod16/1
  dotprod16/1 -> Mux/16
  "IW{1,1}(17,:)'"/1 -> dotprod17/1
  dotprod17/1 -> Mux/17
  "IW{1,1}(18,:)'"/1 -> dotprod18/1
  dotprod18/1 -> Mux/18
  "IW{1,1}(19,:)'"/1 -> dotprod19/1
  dotprod19/1 -> Mux/19
  "IW{1,1}(20,:)'"/1 -> dotprod20/1
  dotprod20/1 -> Mux/20
  "IW{1,1}(21,:)'"/1 -> dotprod21/1
  dotprod21/1 -> Mux/21
  "IW{1,1}(22,:)'"/1 -> dotprod22/1
  dotprod22/1 -> Mux/22
  "IW{1,1}(23,:)'"/1 -> dotprod23/1
  dotprod23/1 -> Mux/23
  "IW{1,1}(24,:)'"/1 -> dotprod24/1
  dotprod24/1 -> Mux/24
  "IW{1,1}(25,:)'"/1 -> dotprod25/1
  dotprod25/1 -> Mux/25
  "IW{1,1}(26,:)'"/1 -> dotprod26/1
  dotprod26/1 -> Mux/26
  "IW{1,1}(27,:)'"/1 -> dotprod27/1
  dotprod27/1 -> Mux/27
  "IW{1,1}(28,:)'"/1 -> dotprod28/1
  dotprod28/1 -> Mux/28
  "IW{1,1}(29,:)'"/1 -> dotprod29/1
  dotprod29/1 -> Mux/29
  "IW{1,1}(30,:)'"/1 -> dotprod30/1
  dotprod30/1 -> Mux/30
  "IW{1,1}(31,:)'"/1 -> dotprod31/1
  dotprod31/1 -> Mux/31
  "IW{1,1}(32,:)'"/1 -> dotprod32/1
  dotprod32/1 -> Mux/32
  "IW{1,1}(33,:)'"/1 -> dotprod33/1
  dotprod33/1 -> Mux/33
  "IW{1,1}(34,:)'"/1 -> dotprod34/1
  dotprod34/1 -> Mux/34
  "IW{1,1}(35,:)'"/1 -> dotprod35/1
  dotprod35/1 -> Mux/35
  "IW{1,1}(36,:)'"/1 -> dotprod36/1
  dotprod36/1 -> Mux/36
  "IW{1,1}(37,:)'"/1 -> dotprod37/1
  dotprod37/1 -> Mux/37
  "IW{1,1}(38,:)'"/1 -> dotprod38/1
  dotprod38/1 -> Mux/38
  "IW{1,1}(39,:)'"/1 -> dotprod39/1
  dotprod39/1 -> Mux/39
  "IW{1,1}(40,:)'"/1 -> dotprod40/1
  dotprod40/1 -> Mux/40
  Mux/1 -> "iz{1,1}"/1

== system mrefrobotarm_modified_previous_y_previous_u_previous_ref_Thao/cex_3_part/Layer 2/Delays 1 ==
  "p{2}" : Inport  PortDimensions=40
      mask Display: e = 0.06;c1 = [120 230 180]/255;c2 = ([120 230 180]+0)/(256+128);c3 = ([120 230 180]+128)/(256+128);patch([0 1 1 0],[0 0 1 1],c1);patch([0 1 1 1-e 1-e 0+e],[0 0 1 1-e 0+e 0+e],c2);patch([0 0 1 1-e 0+e 0+e],[0 1 1 1-e 1-e 0+e],c3);plot([0 1 1 0 0],[0 0 1 1 0]);
  mux : Mux  Inputs=1
      mask Display: e = 0.06;c1 = [120 150 230]/255;c2 = ([120 150 230]+0)/383;c3 = ([120 150 230]+128)/383;patch([0 1 1 0],[0 0 1 1],c1);patch([0 1 1 1-e 1-e 0+e],[0 0 1 1-e 0+e 0+e],c2);patch([0 0 1 1-e 0+e 0+e],[0 1 1 1-e 1-e 0+e],c3);plot([0 1 1 0 0],[0 0 1 1 0]);disp('Mux')
  "pd{2,1}" : Outport
      mask Display: e = 0.06;c1 = [120 230 180]/255;c2 = ([120 230 180]+0)/(256+128);c3 = ([120 230 180]+128)/(256+128);patch([0 1 1 0],[0 0 1 1],c1);patch([0 1 1 1-e 1-e 0+e],[0 0 1 1-e 0+e 0+e],c2);patch([0 0 1 1-e 0+e 0+e],[0 1 1 1-e 1-e 0+e],c3);plot([0 1 1 0 0],[0 0 1 1 0]);
  wires:
  "p{2}"/1 -> mux/1
  mux/1 -> "pd{2,1}"/1

== system mrefrobotarm_modified_previous_y_previous_u_previous_ref_Thao/cex_3_part/Layer 2/LW{2,1} ==
  "ad{2,1}" : Inport  PortDimensions=40
      mask Display: e = 0.06;c1 = [120 230 180]/255;c2 = ([120 230 180]+0)/(256+128);c3 = ([120 230 180]+128)/(256+128);patch([0 1 1 0],[0 0 1 1],c1);patch([0 1 1 1-e 1-e 0+e],[0 0 1 1-e 0+e 0+e],c2);patch([0 0 1 1-e 0+e 0+e],[0 1 1 1-e 1-e 0+e],c3);plot([0 1 1 0 0],[0 0 1 1 0]);
  "IW{2,1}(1,:)'" : Constant  Value=[-0.2110296507689225220527617921106866560876369476318359375;0.129194370492478227685495539844851009547710418701171875;0.8478328949031437300476454765885137021541595458984375;0.59311399751551163728180426915059797465801239013671875;0.374472612428015716456997097338899038732051849365234375;0.0770615628520603113127407368665444664657115936279296875;0.353819585433120697981479452209896408021450042724609375;0.10512816289559910598594427710850141011178493499755859375;-0.274664423972334592605193392955698072910308837890625;0.317908678194257443561099307771655730903148651123046875;0.2916331476774314257482956236344762146472930908203125;-0.154232625574055204342727165567339397966861724853515625;0.4606225905632814754397941214847378432750701904296875;0.449352051449551037620722127030603587627410888671875;0.38192972830325311317523073739721439778804779052734375;0.198758909060646471456124118049046956002712249755859375;-0.188625455594572055684210454273852519690990447998046875;0.3405987413390183515815579085028730332851409912109375;-0.31139327029567454019343131221830844879150390625;0.26999016589972890667326055336161516606807708740234375;-0.0561884207933089907527346440474502742290496826171875;0.276744113814034686793519313141587190330028533935546875;0.173646500083200316932874329722835682332515716552734375;0.24631630195219422763130978637491352856159210205078125;0.193023660131389274141611167578957974910736083984375;-0.39352911655069167107257044335710816085338592529296875;-0.237547740730999767944098266525543294847011566162109375;-0.095622343523369790485588737283251248300075531005859375;0.04926355729475236089331957600734313018620014190673828125;0.41616634819587527971407325821928679943084716796875;-0.20578282407495052108714617133955471217632293701171875;-0.2462199213135418951470256843094830401241779327392578125;-0.1187439439471112689883369739618501625955104827880859375;0.042220266895537213180933377998371724970638751983642578125;-0.310983644648225421303067150802235119044780731201171875;-0.27230526456576609195536775587243027985095977783203125;0.008753961429150462769666063422846491448581218719482421875;-0.152171624528346594029670768577489070594310760498046875;0.236014894049587142799140337956487201154232025146484375;0.7796541310705009664161480031907558441162109375]
      mask Display: e = 0.06;c1 = [120 150 230]/255;c2 = ([120 150 230]+0)/383;c3 = ([120 150 230]+128)/383;patch([0 1 1 0],[0 0 1 1],c1);patch([0 1 1 1-e 1-e 0+e],[0 0 1 1-e 0+e 0+e],c2);patch([0 0 1 1-e 0+e 0+e],[0 1 1 1-e 1-e 0+e],c3);plot([0 1 1 0 0],[0 0 1 1 0]);disp('weights');
  Mux : Mux  Inputs=1
      mask Display: e = 0.06;c1 = [120 150 230]/255;c2 = ([120 150 230]+0)/383;c3 = ([120 150 230]+128)/383;patch([0 1 1 0],[0 0 1 1],c1);patch([0 1 1 1-e 1-e 0+e],[0 0 1 1-e 0+e 0+e],c2);patch([0 0 1 1-e 0+e 0+e],[0 1 1 1-e 1-e 0+e],c3);plot([0 1 1 0 0],[0 0 1 1 0]);disp('Mux');
  dotprod1 : neural/Weight Functions/dotprod
  "lz{2,1}" : Outport
      mask Display: e = 0.06;c1 = [120 230 180]/255;c2 = ([120 230 180]+0)/(256+128);c3 = ([120 230 180]+128)/(256+128);patch([0 1 1 0],[0 0 1 1],c1);patch([0 1 1 1-e 1-e 0+e],[0 0 1 1-e 0+e 0+e],c2);patch([0 0 1 1-e 0+e 0+e],[0 1 1 1-e 1-e 0+e],c3);plot([0 1 1 0 0],[0 0 1 1 0]);
  wires:
  "IW{2,1}(1,:)'"/1 -> dotprod1/1
  "ad{2,1}"/1 -> dotprod1/2
  dotprod1/1 -> Mux/1
  Mux/1 -> "lz{2,1}"/1

== system mrefrobotarm_modified_previous_y_previous_u_previous_ref_Thao/good_one/Layer 1/Delays 1 ==
  "p{1}" : Inport  PortDimensions=10
      mask Display: e = 0.06;c1 = [120 230 180]/255;c2 = ([120 230 180]+0)/(256+128);c3 = ([120 230 180]+128)/(256+128);patch([0 1 1 0],[0 0 1 1],c1);patch([0 1 1 1-e 1-e 0+e],[0 0 1 1-e 0+e 0+e],c2);patch([0 0 1 1-e 0+e 0+e],[0 1 1 1-e 1-e 0+e],c3);plot([0 1 1 0 0],[0 0 1 1 0]);
  mux : Mux  Inputs=1
      mask Display: e = 0.06;c1 = [120 150 230]/255;c2 = ([120 150 230]+0)/383;c3 = ([120 150 230]+128)/383;patch([0 1 1 0],[0 0 1 1],c1);patch([0 1 1 1-e 1-e 0+e],[0 0 1 1-e 0+e 0+e],c2);patch([0 0 1 1-e 0+e 0+e],[0 1 1 1-e 1-e 0+e],c3);plot([0 1 1 0 0],[0 0 1 1 0]);disp('Mux')
  "pd{1,1}" : Outport
      mask Display: e = 0.06;c1 = [120 230 180]/255;c2 = ([120 230 180]+0)/(256+128);c3 = ([120 230 180]+128)/(256+128);patch([0 1 1 0],[0 0 1 1],c1);patch([0 1 1 1-e 1-e 0+e],[0 0 1 1-e 0+e 0+e],c2);patch([0 0 1 1-e 0+e 0+e],[0 1 1 1-e 1-e 0+e],c3);plot([0 1 1 0 0],[0 0 1 1 0]);
  wires:
  "p{1}"/1 -> mux/1
  mux/1 -> "pd{1,1}"/1
